simulink model "Prob_7_Oral_Metformin-3 (1)"  (R2024b)
settings: Solver=VariableStepAuto  StartTime=0.0  StopTime=24  RelTol=1e-3
settings Model: Creator=claudelieber  LastModifiedBy=claudelieber
settings RTWCC: GPUComputeCapability=3.5

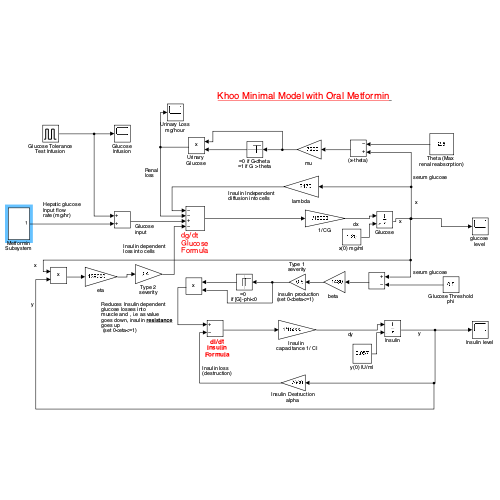
[thumbnail: Simulink's stored preview of the top-level diagram]
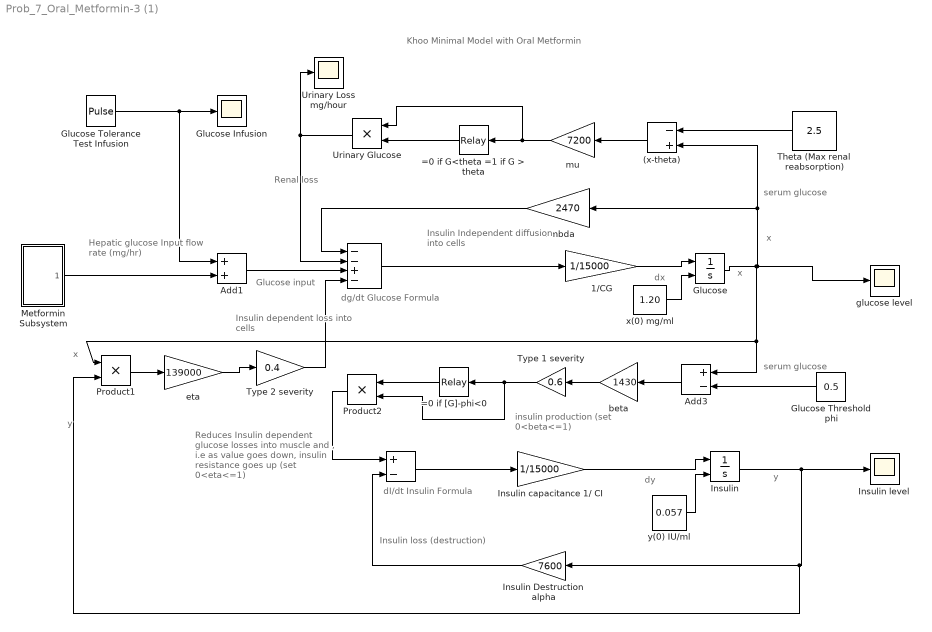
== system Prob_7_Oral_Metformin-3 (1) ==
  note: Khoo Minimal Model with Oral Metformin
  note: insulin production
      | (set 0<beta<=1)
  note: serum glucose
  note: Insulin dependent
      | loss into cells
  note: dI/dt
      | Insulin
      | Formula
  note: y
  note: Hepatic glucose
      | Input flow
      | rate (mg/hr)
  note: serum glucose
  note: dg/dt
      | Glucose
      | Formula
  note: Insulin loss
      | (destruction)
  note: x
  note: Reduces Insulin dependent
      | glucose losses into
      | muscle and , i.e as value
      | goes down, insulin resistance
      | goes up
      | (set 0<eta<=1)
  note: Glucose
      | input
  note: dx
  note: dy
  note: y
  note: x
  note: x
  note: Insulin Independent
      | diffusion into cells
  note: Renal
      | loss
  " " : Sum  Inputs=--+-
  " " : Sum  Inputs=+-
  (x-theta) : Sum  Inputs=-+
  1/CG : Gain  Gain=1/15000
  =0 if [G]-phi<0 : Relay  OnSwitchValue=0  OffSwitchValue=-0.0001
  =0 if G<theta =1 if G > theta : Relay  OnSwitchValue=0  OffSwitchValue=-0.00001
  Add1 : Sum
  Add3 : Sum  Inputs=+-
  Glucose : Integrator  InitialConditionSource=external  InitialCondition=0.81
  Glucose Infusion : Scope
  Glucose Threshold phi : Constant  Value=0.5
  Glucose Tolerance Test Infusion : DiscretePulseGenerator  PulseType=Time based  Amplitude=0  Period=10  PulseWidth=5
  Insulin : Integrator  InitialConditionSource=external  InitialCondition=0.055
  Insulin capacitance 1/ CI : Gain  Gain=1/15000
  Insulin Destruction alpha : Gain  Gain=7600
  Insulin level : Scope
  Metformin Subsystem : Subsystem
  Product1 : Product
  Product2 : Product
  Theta (Max renal reabsorption) : Constant  Value=2.5
  Type 1 severity : Gain  Gain=0.6
  Type 2 severity : Gain  Gain=0.4
  Urinary Glucose : Product
  Urinary Loss mg/hour : Scope
  "beta " : Gain  Gain=1430
  "eta " : Gain  Gain=139000
  glucose level : Scope
  lambda : Gain  Gain=2470
  mu : Gain  Gain=7200
  x(0) mg/ml : Constant  Value=1.20
  y(0) IU/ml : Constant  Value=0.057
  wires:
  "beta "/1 -> Type 1 severity/1
  Glucose/1 -> Product1/1, Add3/1, glucose level/1, (x-theta)/2, lambda/1
  (x-theta)/1 -> mu/1
  " "/1 -> 1/CG/1
  Product2/1 -> " "/1
  Add3/1 -> "beta "/1
  lambda/1 -> " "/1
  Insulin capacitance 1/ CI/1 -> Insulin/1
  "eta "/1 -> Type 2 severity/1
  x(0) mg/ml/1 -> Glucose/2
  1/CG/1 -> Glucose/1
  Metformin Subsystem/1(Output) -> Add1/2
  =0 if G<theta =1 if G > theta/1 -> Urinary Glucose/2
  =0 if [G]-phi<0/1 -> Product2/1
  Add1/1 -> " "/3
  " "/1 -> Insulin capacitance 1/ CI/1
  Glucose Tolerance Test Infusion/1 -> Add1/1, Glucose Infusion/1
  Type 2 severity/1 -> " "/4
  y(0) IU/ml/1 -> Insulin/2
  Insulin Destruction alpha/1 -> " "/2
  Product1/1 -> "eta "/1
  Type 1 severity/1 -> Product2/2, =0 if [G]-phi<0/1
  mu/1 -> Urinary Glucose/1, =0 if G<theta =1 if G > theta/1
  Theta (Max renal reabsorption)/1 -> (x-theta)/1
  Glucose Threshold phi/1 -> Add3/2
  Insulin/1 -> Product1/2, Insulin Destruction alpha/1, Insulin level/1
  Urinary Glucose/1 -> " "/2, Urinary Loss mg/hour/1

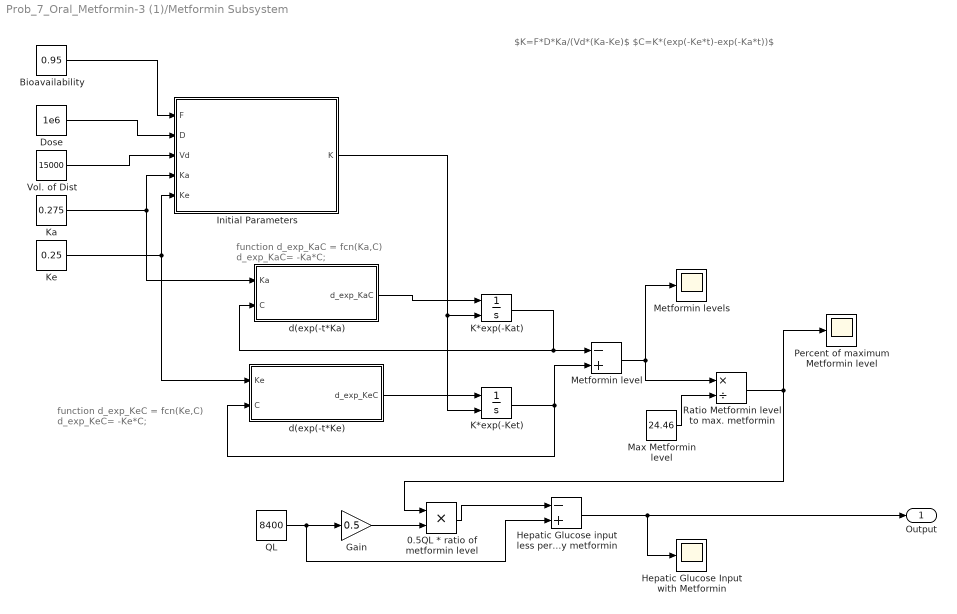
== system Prob_7_Oral_Metformin-3 (1)/Metformin Subsystem ==
  note: function d_exp_KeC = fcn(Ke,C)
      | d_exp_KeC= -Ke*C;
  note: $K=F*D*Ka/(Vd*(Ka-Ke)$
      | $C=K*(exp(-Ke*t)-exp(-Ka*t))$
  note: function d_exp_KaC = fcn(Ka,C)
      | d_exp_KaC= -Ka*C;
  0.5QL * ratio of metformin level : Product
  Bioavailability : Constant  Value=0.95
  Dose : Constant  Value=1e6
  Gain : Gain  Gain=0.5
  Hepatic Glucose Input with Metformin : Scope
  Hepatic Glucose input less percent suppressed by metformin : Sum  Inputs=-+
  Initial Parameters : MATLAB Function  TreatAsAtomicUnit=on
  K*exp(-Kat) : Integrator  InitialConditionSource=external
  K*exp(-Ket) : Integrator  InitialConditionSource=external
  Ka : Constant  Value=0.275
  Ke : Constant  Value=0.25
  Max Metformin level : Constant  Value=24.46
  Metformin level : Sum  Inputs=-+
  Metformin levels : Scope
  Percent of maximum Metformin level : Scope
  QL : Constant  Value=8400
  Ratio Metformin level to max. metformin : Product  Inputs=*/
  Vol. of Dist : Constant  Value=15000
  d(exp(-t*Ka) : MATLAB Function  TreatAsAtomicUnit=on
  d(exp(-t*Ke) : MATLAB Function  TreatAsAtomicUnit=on
  Output : Outport
  wires:
  Max Metformin level/1 -> Ratio Metformin level to max. metformin/2
  Gain/1 -> 0.5QL * ratio of metformin level/2
  Vol. of Dist/1 -> Initial Parameters/3(Vd)
  Initial Parameters/1(K) -> K*exp(-Kat)/2, K*exp(-Ket)/2
  Bioavailability/1 -> Initial Parameters/1(F)
  Dose/1 -> Initial Parameters/2(D)
  QL/1 -> Hepatic Glucose input less percent suppressed by metformin/2, Gain/1
  Ratio Metformin level to max. metformin/1 -> Percent of maximum Metformin level/1, 0.5QL * ratio of metformin level/1
  d(exp(-t*Ke)/1(d_exp_KeC) -> K*exp(-Ket)/1
  K*exp(-Ket)/1 -> d(exp(-t*Ke)/2(C), Metformin level/2
  Hepatic Glucose input less percent suppressed by metformin/1 -> Output/1, Hepatic Glucose Input with Metformin/1
  Metformin level/1 -> Ratio Metformin level to max. metformin/1, Metformin levels/1
  Ke/1 -> d(exp(-t*Ke)/1(Ke), Initial Parameters/5(Ke)
  0.5QL * ratio of metformin level/1 -> Hepatic Glucose input less percent suppressed by metformin/1
  K*exp(-Kat)/1 -> Metformin level/1, d(exp(-t*Ka)/2(C)
  Ka/1 -> d(exp(-t*Ka)/1(Ka), Initial Parameters/4(Ka)
  d(exp(-t*Ka)/1(d_exp_KaC) -> K*exp(-Kat)/1

== matlab function Prob_7_Oral_Metformin-3 (1)/Metformin Subsystem/d(exp(-t*Ke) ==
  data: Ke input; d_exp_KeC output; C input
function d_exp_KeC = fcn(Ke,C)

d_exp_KeC= -Ke*C;

== matlab function Prob_7_Oral_Metformin-3 (1)/Metformin Subsystem/Initial Parameters ==
  data: F input; K output; D input; Vd input; Ka input; Ke input
function K = fcn(F,D,Vd,Ka,Ke)

K = F*D*Ka/(Vd*(Ka-Ke));

== matlab function Prob_7_Oral_Metformin-3 (1)/Metformin Subsystem/d(exp(-t*Ka) ==
  data: Ka input; d_exp_KaC output; C input
function d_exp_KaC = fcn(Ka,C)
d_exp_KaC= -Ka*C;
